simulink model "rf_system"  (R2022b)
settings: Solver=VariableStepAuto  StartTime=0.0  StopTime=10.0  RelTol=1e-3
PreLoadFcn:
  | clear;
  | 
  | sample_time=1/116e6;
  | carriers.LO = 22e9;
  | carriers.LOL = carriers.LO/2;
  | carriers.LOH = carriers.LO*3;
  | carriers.OUT = carriers.LO*3.5;
  | 
  | %Put all carriers in one vector for convenience
  | car_env = unique(structfun(@deal,carriers));
  | 
  | 
  | % Lower limit of frequency (governed by impulse duration):
  | Duration = sample_time*128;
  | LLFreq = 1/Duration;
  | 
  | 
  | %Upper limit of frequency (governed by sample time):
  | ULFreq = 1/(2*sample_time);
  | 
  | 
  | % Generate 1/f phase noise with -60dBc/Hz level @ 1KHz:
  | PhNoOffsets = [LLFreq 1e3 ULFreq];
  | PhNoLevels = -40-10*log10(PhNoOffsets/1e3);
libraries: simrfV2util1 x7, dspstat3 x5, simrfV2sources1 x2, simrfV2elements x1, simulink x1
settings Model: SimulationMode=accelerator  Creator=hessam  LastModifiedBy=hessam

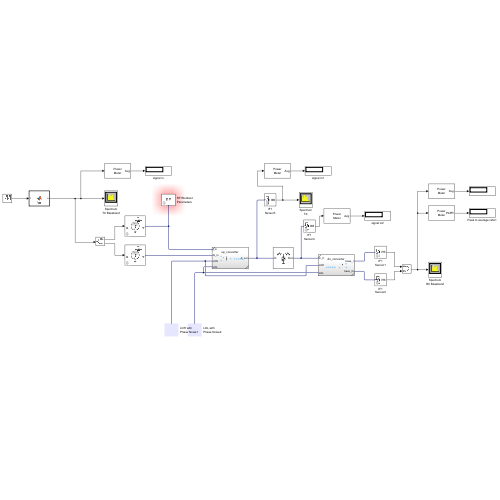
[thumbnail: Simulink's stored preview of the top-level diagram]
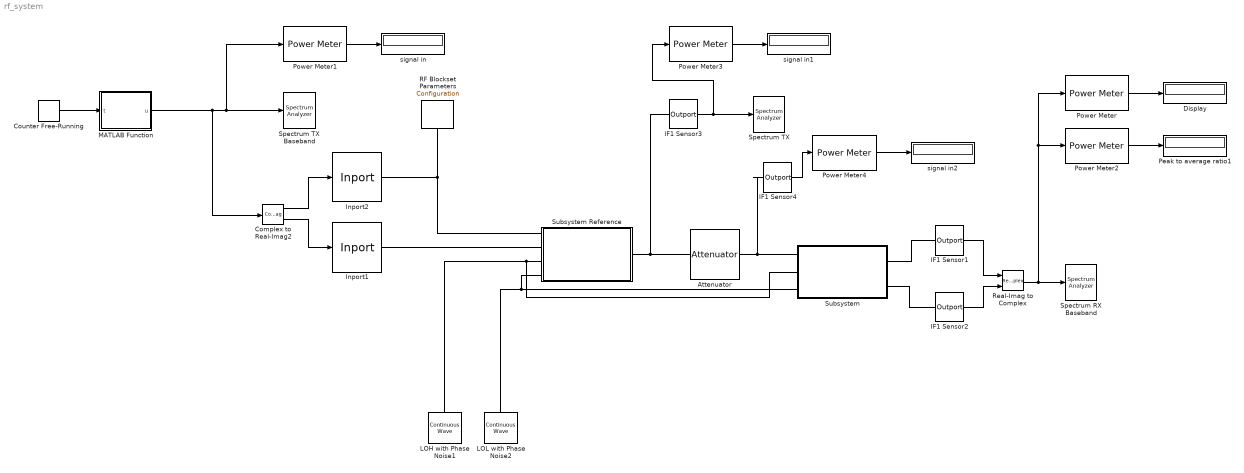
== system rf_system ==
  Attenuator : simrfV2elements/Attenuator  classname=attenuator  Att=30  Zin=50  Zout=50  AddNoise=on  InternalGrounding=on
  Complex to Real-Imag2 : ComplexToRealImag
  Counter Free-Running : simulink/Sources/Counter Free-Running  NumBits=24  tsamp=-1
  Display : Display
  IF1 Sensor1 : simrfV2util1/Outport  SensorType=Power  OutputFormat=Real Passband  CarrierFreq=0 Hz  ZL=50  InternalGrounding=on  StepSize=-1 s  AutoStep=off
  IF1 Sensor2 : simrfV2util1/Outport  SensorType=Power  OutputFormat=Real Passband  CarrierFreq=0 Hz  ZL=50  InternalGrounding=on  StepSize=-1 s  AutoStep=off
  IF1 Sensor3 : simrfV2util1/Outport  SensorType=Power  OutputFormat=Complex Baseband  CarrierFreq=carriers.OUT Hz  ZL=50  InternalGrounding=on  StepSize=-1 s  AutoStep=off
  IF1 Sensor4 : simrfV2util1/Outport  SensorType=Power  OutputFormat=Complex Baseband  CarrierFreq=carriers.OUT Hz  ZL=50  InternalGrounding=on  StepSize=-1 s  AutoStep=off
  Inport1 : simrfV2util1/Inport  SimulinkInputSignalType=Power  CarrierFreq=0 Hz  ZS=50  UseSqWave=off  NumCoeff=10  Bias=0  DutyCyc=50  InternalGrounding=on
  Inport2 : simrfV2util1/Inport  SimulinkInputSignalType=Power  CarrierFreq=0 Hz  ZS=50  UseSqWave=off  NumCoeff=10  Bias=0  DutyCyc=50  InternalGrounding=on
  LOH with Phase Noise1 : simrfV2sources1/Continuous Wave  CWSourceType=Ideal voltage  Z0=0  IVoltage=1 V  ICurrent=0 A  MagPower=0 W  QVoltage=0 V  QCurrent=0 A  AnglePower=0  CarrierFreq=carriers.LOH Hz  AddPhaseNoise=off  PhaseNoiseOffset=PhNoOffsets  PhaseNoiseLevel=PhNoLevels  AutoImpulseLength=on  ImpulseLength=1e-10 s  InternalGrounding=on
  LOL with Phase Noise2 : simrfV2sources1/Continuous Wave  CWSourceType=Ideal voltage  Z0=0  IVoltage=1 V  ICurrent=0 A  MagPower=0 W  QVoltage=0 V  QCurrent=0 A  AnglePower=0  CarrierFreq=carriers.LOL Hz  AddPhaseNoise=on  PhaseNoiseOffset=PhNoOffsets  PhaseNoiseLevel=PhNoLevels  AutoImpulseLength=on  ImpulseLength=1e-10 s  InternalGrounding=on
  MATLAB Function : MATLAB Function  TreatAsAtomicUnit=on
  Peak to average ratio1 : Display
  Power Meter : dspstat3/Power Meter  Measurement=Average power  ReferenceLoad=1  OutputPowerUnits=dBm  WindowLength=1024  OverlapLength=1023  AllowArbitraryInputLength=on  ComputeCCDF=off  PowerRange=50  PowerResolution=0.1  CCDFOutput=Relative power (dB above average power)  ProbabilityVector=[ 10; 1; 0.1; 0.01; 0.001; 0.0001 ]  RelativePowerVector=[ 0; 3; 6; 9; 12 ]  ResetPort=off  SimulateUsing=Code generation
      settings: LibrarySourceBlock=commutil2/Power Meter
  Power Meter1 : dspstat3/Power Meter  Measurement=Average power  ReferenceLoad=1  OutputPowerUnits=dBm  WindowLength=256  OverlapLength=255  AllowArbitraryInputLength=on  ComputeCCDF=off  PowerRange=50  PowerResolution=0.1  CCDFOutput=Relative power (dB above average power)  ProbabilityVector=[ 10; 1; 0.1; 0.01; 0.001; 0.0001 ]  RelativePowerVector=[ 0; 3; 6; 9; 12 ]  ResetPort=off  SimulateUsing=Code generation
      settings: LibrarySourceBlock=commutil2/Power Meter
  Power Meter2 : dspstat3/Power Meter  Measurement=Peak-to-average power ratio  ReferenceLoad=1  OutputPowerUnits=dBm  WindowLength=256  OverlapLength=255  AllowArbitraryInputLength=on  ComputeCCDF=off  PowerRange=50  PowerResolution=0.1  CCDFOutput=Relative power (dB above average power)  ProbabilityVector=[ 10; 1; 0.1; 0.01; 0.001; 0.0001 ]  RelativePowerVector=[ 0; 3; 6; 9; 12 ]  ResetPort=off  SimulateUsing=Code generation
      settings: LibrarySourceBlock=commutil2/Power Meter
  Power Meter3 : dspstat3/Power Meter  Measurement=Average power  ReferenceLoad=1  OutputPowerUnits=dBm  WindowLength=256  OverlapLength=255  AllowArbitraryInputLength=on  ComputeCCDF=off  PowerRange=50  PowerResolution=0.1  CCDFOutput=Relative power (dB above average power)  ProbabilityVector=[ 10; 1; 0.1; 0.01; 0.001; 0.0001 ]  RelativePowerVector=[ 0; 3; 6; 9; 12 ]  ResetPort=off  SimulateUsing=Code generation
      settings: LibrarySourceBlock=commutil2/Power Meter
  Power Meter4 : dspstat3/Power Meter  Measurement=Average power  ReferenceLoad=1  OutputPowerUnits=dBm  WindowLength=256  OverlapLength=255  AllowArbitraryInputLength=on  ComputeCCDF=off  PowerRange=50  PowerResolution=0.1  CCDFOutput=Relative power (dB above average power)  ProbabilityVector=[ 10; 1; 0.1; 0.01; 0.001; 0.0001 ]  RelativePowerVector=[ 0; 3; 6; 9; 12 ]  ResetPort=off  SimulateUsing=Code generation
      settings: LibrarySourceBlock=commutil2/Power Meter
  RF Blockset Parameters : simrfV2util1/Configuration  AutoFreq=on  Tones="[11  66] GHz"  Harmonics="[5  5]"  NormalizeCarrierPower=on  SolverType=Auto  UseCCode=on  StepSize=sample_time s  AddNoise=off  defaultRNG=on  Seed=0  Temperature=293.15 K  SolverDelFlag=0  AbsTol=1e-6  RelTol=1e-3  MaxIter=10  ErrorEstimationType=2-norm over all variables  EnableInterpFilter=off  HiddenFIRfilterControllerParam=off  SmallSignalApprox=off  AllSimFreqs=on  SimFreqs=[] Hz  SimFreqsInternal=[]  SamplesPerFrame=1
  Real-Imag to Complex : RealImagToComplex
  Spectrum RX Baseband : SpectrumAnalyzer
  Spectrum TX : SpectrumAnalyzer
  Spectrum TX Baseband : SpectrumAnalyzer
  Subsystem : Subsystem  ReferencedSubsystem=dn_converter
      settings: PortSchema="{\"entries\":[{\"content\":{\"sides\":[{\"content\":{\"connectorIds\":[\"LConn3\",\"LConn1\",\"LConn2\"]},\"type\":\"ConnectorPlacement.EquallySpacedRectSide\",\"uuid\":\"8336b51e-e5d8-49cc-804f-7bfb99400ab0\"},{\"content\":{\"connectorIds\":[\"LConn4\",\"LConn5\"],\"side\":\"RIGHT\"},\"type\":\"ConnectorPlacement.EquallySpacedRectSide\",\"uuid\":\"6f005c77-3014-47d2-89f9-41814728faba\"},{\"content\":{\"connectorIds\":[],\"side\":\"TOP\"},\"type\":\"ConnectorPlacement.EquallySpacedRectSide\",\"uuid\":\"edcdef5b-1b73-4458-84fc-72d761e40cdf\"}]},\"type\":\"ConnectorPlacement.EquallySpacedConnector\",\"uuid\":\"3f0b5c66-2f3f-40e5-bb1c-488293219f70\"}],\"packageUris\":[\"http://schema.mathworks.com/mf0/Connector/R2020b\"],\"version\":\"1.0\"}"
  Subsystem Reference : Subsystem  ReferencedSubsystem=up_converter
      settings: PortSchema="{\"entries\":[{\"content\":{\"sides\":[{\"content\":{\"connectorIds\":[\"LConn3\",\"LConn4\",\"LConn2\",\"LConn1\"]},\"type\":\"ConnectorPlacement.EquallySpacedRectSide\",\"uuid\":\"8336b51e-e5d8-49cc-804f-7bfb99400ab0\"},{\"content\":{\"connectorIds\":[\"LConn5\"],\"side\":\"RIGHT\"},\"type\":\"ConnectorPlacement.EquallySpacedRectSide\",\"uuid\":\"6f005c77-3014-47d2-89f9-41814728faba\"},{\"content\":{\"connectorIds\":[],\"side\":\"TOP\"},\"type\":\"ConnectorPlacement.EquallySpacedRectSide\",\"uuid\":\"edcdef5b-1b73-4458-84fc-72d761e40cdf\"}]},\"type\":\"ConnectorPlacement.EquallySpacedConnector\",\"uuid\":\"3f0b5c66-2f3f-40e5-bb1c-488293219f70\"}],\"packageUris\":[\"http://schema.mathworks.com/mf0/Connector/R2020b\"],\"version\":\"1.0\"}"
  signal in : Display
  signal in1 : Display
  signal in2 : Display
  wires:
  Counter Free-Running/1 -> MATLAB Function/1(t)
  Power Meter1/1 -> signal in/1
  MATLAB Function/1(u) -> Complex to Real-Imag2/1, Spectrum TX Baseband/1, Power Meter1/1
  Complex to Real-Imag2/1 -> Inport2/1
  Complex to Real-Imag2/2 -> Inport1/1
  IF1 Sensor1/1 -> Real-Imag to Complex/1
  Power Meter/1 -> Display/1
  Real-Imag to Complex/1 -> Power Meter2/1, Power Meter/1, Spectrum RX Baseband/1
  Power Meter2/1 -> Peak to average ratio1/1
  IF1 Sensor2/1 -> Real-Imag to Complex/2
  IF1 Sensor3/1 -> Power Meter3/1, Spectrum TX/1
  Power Meter3/1 -> signal in1/1
  Power Meter4/1 -> signal in2/1
  IF1 Sensor4/1 -> Power Meter4/1
  connections:
  Subsystem Reference/LConn5 -- IF1 Sensor3/LConn1 -- Attenuator/LConn1
  Subsystem/LConn3 -- IF1 Sensor4/LConn1 -- Attenuator/RConn1
  Subsystem/LConn1 -- LOH with Phase Noise1/LConn1 -- Subsystem Reference/LConn2
  LOL with Phase Noise2/LConn1 -- Subsystem/LConn2 -- Subsystem Reference/LConn1
  RF Blockset Parameters/LConn1 -- Subsystem Reference/LConn3 -- Inport2/RConn1
  Subsystem Reference/LConn4 -- Inport1/RConn1
  Subsystem/LConn5 -- IF1 Sensor2/LConn1
  Subsystem/LConn4 -- IF1 Sensor1/LConn1

== matlab function rf_system/MATLAB Function ==
  data: u output; t input
function u   = fcn(t)
   %test of the block
   t=double(t);
   pdb=-16;   %dial input power in dBm 50-ohm reference
   v = sqrt(1/1000*10^(pdb/10));
   f=[1 2 3 4 5 6  ]*455e-5;
   u=v*sum(exp(2.0*3.14*f*t*1j));
